simulink subsystem "bicycle"  (R2022b)
settings: Solver=VariableStepAuto  StartTime=0.0  StopTime=10.0  RelTol=1e-3
values from neighbouring files (symbols this model uses):
  g = 9.81    [gyro_and_bicycle_params.m]
  k1 = Ibz + mb*hb^2 + mf*hf^2 + (Ifz + Ifx + 2*mf*hf^2) + mg*hg^2 +(Igz + Igx + 2*mg*hg^2)    (= 20.1934)    [gyro_and_bicycle_params.m]
  k2 = mb*hb + mf*hf + mg*hg    (= 17.89)    [gyro_and_bicycle_params.m]
settings Model: Creator=baran  LastModifiedBy=baran

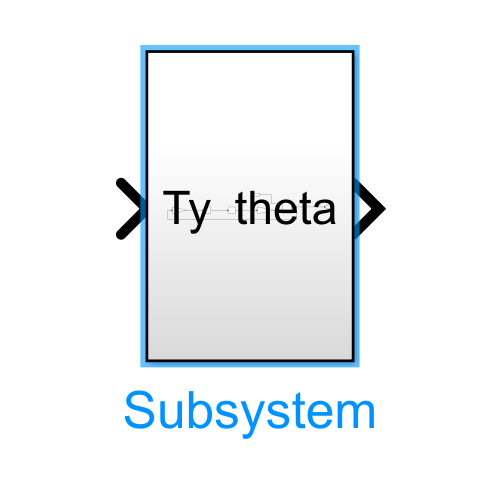
[thumbnail: Simulink's stored preview of the top-level diagram]
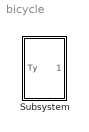
== system bicycle ==
  Subsystem : Subsystem

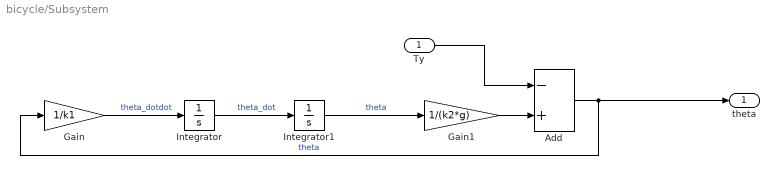
== system bicycle/Subsystem ==
  Ty : Inport
  Add : Sum  Inputs=-+
  Gain : Gain  Gain=1/k1
  Gain1 : Gain  Gain=1/(k2*g)
  Integrator : Integrator
  Integrator1 : Integrator
  theta : Outport
  wires:
  Ty/1 -> Add/1
  Integrator/1 -> Integrator1/1  "theta_dot"
  Gain/1 -> Integrator/1  "theta_dotdot"
  Add/1 -> theta/1, Gain/1  "theta"
  Integrator1/1 -> Gain1/1  "theta"
  Gain1/1 -> Add/2
